simulink model "ConditionActionLoop_2018a"  (R2018a)
settings: Solver=VariableStepAuto  StartTime=0.0  StopTime=10.0  RelTol=1e-3
settings Model: Creator=apple  LastModifiedBy=apple
settings DataIOCC: ReturnWorkspaceOutputs=on
settings SFSimCC: SimUseLocalCustomCode=on
settings RTWCC: RTWUseLocalCustomCode=on

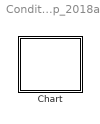
== system ConditionActionLoop_2018a ==
  Chart : Stateflow chart  TreatAsAtomicUnit=on

== stateflow chart ConditionActionLoop_2018a/Chart ==
  state A
    en:fprintf("Entry A");
    du:fprintf("During A");
    ex:fprintf("Exit A");
  state B
    en:fprintf("Entry B");
    du:fprintf("During B");
    ex:fprintf("Exit B");
  (default) -> A
  (junction 3) -> (junction 3) [order 1] : [i<10]{i = i + 1;fprintf('%f',i);}
  A -> (junction 3) : E_one{i = 0}
  (junction 3) -> B [order 2]
  data: i local
  events: E_one local FUNCTION_CALL_EVENT
